simulink model "final63level"  (R2020a)
settings: Solver=ode45  StartTime=0.0  StopTime=.05  RelTol=5e-7  EnableMultiTasking=on
libraries: powerlib x42, re_lib x1, powerlib_meascontrol x1
settings Model: Creator=harish  LastModifiedBy=sunil
settings SolverCC: AlgebraicLoopSolver=LineSearch
settings DataIOCC: LimitDataPoints=on  SaveFormat=Array  ReturnWorkspaceOutputs=off
settings OptimizationCC: LifeSpan=inf
settings DebuggingCC: SFUnexpectedBacktrackingDiag=warning  SFNoUnconditionalDefaultTransitionDiag=warning  SFExecutionAtInitializationDiag=none  ArithmeticOperatorsInVariantConditions=warning
settings HardwareCC: ProdBitPerPointer=32  ProdBitPerSizeT=32  ProdBitPerPtrDiffT=32  ProdLargestAtomicFloat=None  ProdIntDivRoundTo=Undefined  ProdEndianess=Unspecified  ProdWordSize=32  ProdHWDeviceType=32-bit Generic
settings ModelReferenceCC: PropagateSignalLabelsOutOfModel=off
settings SFSimCC: SimUseLocalCustomCode=off  CustomCodeUndefinedFunction=UseInterfaceOnly
settings RTWCC: RTWUseLocalCustomCode=off
settings CodeAppCC: StateflowObjectComments=on
settings GRTTargetCC: TargetLangStandard=C89/C90 (ANSI)
settings ConfigComp: CovMetricSettings=dw  CovHtmlReporting=on  CovSaveCumulativeToWorkspaceVar=on  CovSaveSingleToWorkspaceVar=on  CovExternalEMLEnable=off
settings SimscapeCC: SimscapeNormalizeSystem=off

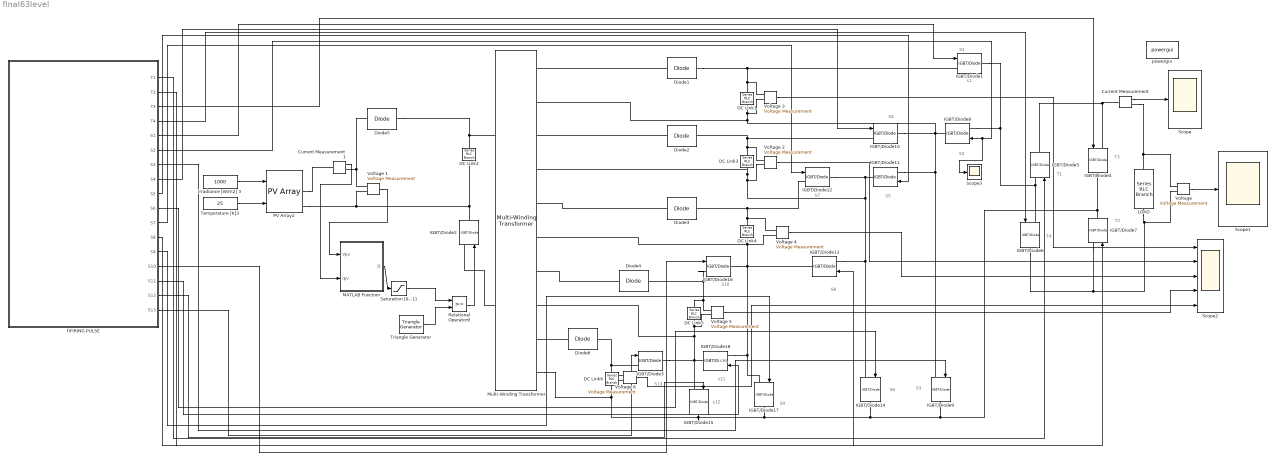
== system final63level ==
  note: s11
  note: s1
  note: S13
  note: s12
  note: s11
  note: S4
  note: S10
  note: S9
  note: S8
  note: S7
  note: S6
  note: S5
  note: S3
  note: S2
  note: S1
  note: T4
  note: T3
  note: T2
  note: T1
  Current Measurement : powerlib/Measurements/Current Measurement  PhasorSimulation=off  OutputType=Complex  PSBequivalent=0
  Current Measurement1 : powerlib/Measurements/Current Measurement  PhasorSimulation=off  OutputType=Complex  PSBequivalent=0
  DC Link1 : powerlib/Elements/Series RLC Branch  LConnTagsString=__new0  RConnTagsString=__new0  BranchType=C  Resistance=1.0  Inductance=1.0  SetiL0=off  InitialCurrent=0  Capacitance=3000e-6  Setx0=off  InitialVoltage=240/31  Measurements=None
      settings: SourceProductBaseCode=MT,PS
  DC Link2 : powerlib/Elements/Series RLC Branch  LConnTagsString=__new0  RConnTagsString=__new0  BranchType=C  Resistance=1.0  Inductance=1.0  SetiL0=off  InitialCurrent=0  Capacitance=300e+6  Setx0=on  InitialVoltage=256  Measurements=None
      settings: SourceProductBaseCode=MT,PS
  DC Link3 : powerlib/Elements/Series RLC Branch  LConnTagsString=__new0  RConnTagsString=__new0  BranchType=C  Resistance=1.0  Inductance=1.0  SetiL0=off  InitialCurrent=0  Capacitance=3000e-6  Setx0=off  InitialVoltage=32  Measurements=None
      settings: SourceProductBaseCode=MT,PS
  DC Link4 : powerlib/Elements/Series RLC Branch  LConnTagsString=__new0  RConnTagsString=__new0  BranchType=C  Resistance=1.0  Inductance=1.0  SetiL0=off  InitialCurrent=0  Capacitance=3000e-6  Setx0=off  InitialVoltage=68  Measurements=None
      settings: SourceProductBaseCode=MT,PS
  DC Link5 : powerlib/Elements/Series RLC Branch  LConnTagsString=__new0  RConnTagsString=__new0  BranchType=C  Resistance=1.0  Inductance=1.0  SetiL0=off  InitialCurrent=0  Capacitance=3000e-6  Setx0=off  InitialVoltage=128  Measurements=None
      settings: SourceProductBaseCode=MT,PS
  DC Link6 : powerlib/Elements/Series RLC Branch  LConnTagsString=__new0  RConnTagsString=__new0  BranchType=C  Resistance=1.0  Inductance=1.0  SetiL0=off  InitialCurrent=0  Capacitance=3000e-6  Setx0=off  InitialVoltage=128  Measurements=None
      settings: SourceProductBaseCode=MT,PS
  Diode{1..6} (6 alike) : powerlib/Power Electronics/Diode  Ron=0.001  Lon=0  Vf=0.8  IC=0  UseSnubber=0  Rs=500  Cs=250e-9  Measurements=off
  IGBT/Diode{1..18} (18 alike) : powerlib/Power Electronics/IGBT//Diode  Ron=1e-3  Rs=1e5  Cs=inf  Measurements=off
  Irradiance [W/m2] 3 : Constant  Value=1000
  LOAD : powerlib/Elements/Series RLC Branch  LConnTagsString=__new0  RConnTagsString=__new0  BranchType=RL  Resistance=250  Inductance=1e-3  SetiL0=off  InitialCurrent=0  Capacitance=1e-6  Setx0=off  InitialVoltage=0  Measurements=None
  MATLAB Function : MATLAB Function  TreatAsAtomicUnit=on
  Multi-Winding Transformer : powerlib/Elements/Multi-Winding Transformer  LeftWindings=1  RightWindings=5  TappedWindings=no taps  NumberOfTaps=4  SetSaturation=off  Hysteresis=off  DataFile='hysteresis.mat'  Measurements=None  UNITS=pu  NominalPower=[1000 10000]  NominalVoltages="[256 240/31   240*2/31   240*4/31  240*8/31  240*16/31]"  WindingResistances=[0 0 0 0 0 0]  WindingInductances="[0 0 0 0 0  0]"  Rm=0.11642  Lm=4.5959e+08  Saturation=[0 0;1.25e-06 1.44e+06;0.00052081 1.824e+06]  BreakLoop=off  DiscreteSolver=Trapezoidal iterative  DataType=off  InitialFlux=0  TransfoNumber=1
      settings: SourceProductBaseCode=PS
  PV Array2 : re_lib/Solar/PV Array  Npar=1  Nser=8  PlotType=array @ 1000 W/m2 & specified temperatures  S_vec="[ 1000  500  100 ]"  Temp_C_vec="[25  ]"  ModuleName=User-defined  PlotWhenSelected=off  Pm=213.15  Ncell=100  Voc=36.3  Isc=7.84  Vm=29  Im=7.35  beta_Voc_pc=-0.36099  alpha_Isc_pc=0.102  beta_Voc=-0.13104  alpha_Isc=0.0079968  IL=7.8541  I0=2.8969e-10  nI=0.58844  Rsh=372.6956  Rs=0.3942  RobustModel=off  RobustCellTemperature=25  BAL=on  Tc=1e-6  Tfilter=5e-5
  Relational Operator9 : RelationalOperator  OutDataTypeStr=boolean  RndMeth=Nearest
  Saturation [0...1] : Saturate  UpperLimit=1  LowerLimit=0
  Scope : Scope
  Scope1 : Scope
  Scope2 : Scope  NumInputPorts=5
  Scope3 : Scope
  Temperature [K]3 : Constant  Value=25
  Triangle Generator : powerlib_meascontrol/Pulse & Signal Generators/Triangle Generator  Freq=1e3  Phase=0  Ts=0
  Voltage {,1..6} (7 alike) : powerlib/Measurements/Voltage Measurement  PhasorSimulation=off  OutputType=Complex  PSBequivalent=0
  fiFIRING PULSE : Subsystem
  powergui : powerlib/powergui  Priority=1  SimulationMode=Discrete  SampleTime=5e-6  frequency=60  Iterations=50  frequencyindice=0  Pbase=100e6  ErrMax=1e-4  UnitsV=kV  UnitsW=MW  buscounter=0  FunctionMessages=off  echomessages=off  EnableUseOfTLC=off  CurrentSourceSwitches=on  DisableSnubberDevices=off  DisableRonSwitches=off  DisableVfSwitches=off  DisplayEquations=off  AutomaticDiscreteSolvers=off  SolverType=Tustin/Backward Euler (TBE)  Interpol=off  ExternalGateDelay=off  methode=off  Ts=100  x0status=blocks  SPID=off  SwTol=0  HookPort=off  NonlinearTolerance=1e-4  nMaxIteration=100  ContinueOnMaxIteration=off  RestoreLinks=warning  ResistiveCurrentMeasurement=off  Frange=[0:2:500]  Ylog=off  Xlog=on  ShowGrid=off  save=off  variable=ZData  structure=load  ZoomFFT=off  StartTime=0.0  cycles=1  DisplayStyle=1  fundamental=50  FreqAxis=on  MaxFrequency=1000  frequencyindicesteady=1  RmsSteady=1  display=off
  wires:
  "Voltage "/1 -> Scope1/1
  Current Measurement/1 -> Scope/1
  fiFIRING PULSE/1(T1) -> IGBT/Diode5/1
  fiFIRING PULSE/2(T2) -> IGBT/Diode7/1
  fiFIRING PULSE/3(T3) -> IGBT/Diode4/1
  fiFIRING PULSE/4(T4) -> IGBT/Diode6/1
  fiFIRING PULSE/5(S1) -> IGBT/Diode1/1
  fiFIRING PULSE/6(S2) -> Scope3/1, IGBT/Diode8/1
  fiFIRING PULSE/7(S3) -> IGBT/Diode9/1
  fiFIRING PULSE/8(S4) -> IGBT/Diode10/1
  fiFIRING PULSE/9(S5) -> IGBT/Diode11/1
  fiFIRING PULSE/10(S6) -> IGBT/Diode14/1
  fiFIRING PULSE/11(S7) -> IGBT/Diode12/1
  fiFIRING PULSE/12(S8) -> IGBT/Diode13/1
  fiFIRING PULSE/13(S9) -> IGBT/Diode17/1
  fiFIRING PULSE/14(S10) -> IGBT/Diode16/1
  MATLAB Function/1(D) -> Saturation [0...1]/1
  Voltage 1/1 -> MATLAB Function/1(Vpv)
  Current Measurement1/1 -> MATLAB Function/2(Ipv)
  Voltage 2/1 -> Scope2/2
  Voltage 3/1 -> Scope2/1
  Voltage 4/1 -> Scope2/3
  Voltage 5/1 -> Scope2/4
  Triangle Generator/1 -> Relational Operator9/2
  Relational Operator9/1 -> IGBT/Diode2/1
  Saturation [0...1]/1 -> Relational Operator9/1
  fiFIRING PULSE/17(S13) -> IGBT/Diode3/1
  fiFIRING PULSE/16(S12) -> IGBT/Diode15/1
  fiFIRING PULSE/15(S11) -> IGBT/Diode18/1
  Voltage 6/1 -> Scope2/5
  Temperature [K]3/1 -> PV Array2/2
  Irradiance [W/m2] 3/1 -> PV Array2/1
  connections:
  IGBT/Diode4/LConn1 -- Current Measurement/LConn1 -- IGBT/Diode5/RConn1
  IGBT/Diode6/LConn1 -- IGBT/Diode8/LConn1 -- IGBT/Diode1/RConn1 -- IGBT/Diode5/LConn1
  "Voltage "/LConn2 -- LOAD/LConn1 -- IGBT/Diode6/RConn1 -- IGBT/Diode7/LConn1
  LOAD/RConn1 -- Current Measurement/RConn1 -- "Voltage "/LConn1
  IGBT/Diode8/RConn1 -- IGBT/Diode10/RConn1 -- IGBT/Diode11/LConn1 -- IGBT/Diode9/LConn1 -- Multi-Winding Transformer/RConn2 -- Voltage 3/LConn2 -- DC Link1/RConn1
  IGBT/Diode12/RConn1 -- IGBT/Diode14/LConn1 -- IGBT/Diode13/LConn1 -- Voltage 2/LConn2 -- DC Link3/RConn1 -- Multi-Winding Transformer/RConn4 -- IGBT/Diode11/RConn1
  IGBT/Diode13/RConn1 -- IGBT/Diode17/LConn1 -- IGBT/Diode18/LConn1 -- IGBT/Diode16/RConn1 -- Voltage 4/LConn2 -- DC Link4/RConn1 -- Multi-Winding Transformer/RConn6
  Voltage 5/LConn2 -- IGBT/Diode3/RConn1 -- IGBT/Diode15/LConn1 -- IGBT/Diode18/RConn1 -- Multi-Winding Transformer/RConn8 -- DC Link5/RConn1
  DC Link1/LConn1 -- IGBT/Diode1/LConn1 -- Diode1/RConn1 -- Voltage 3/LConn1
  Diode1/LConn1 -- Multi-Winding Transformer/RConn1
  Diode2/LConn1 -- Multi-Winding Transformer/RConn3
  Diode3/LConn1 -- Multi-Winding Transformer/RConn5
  Diode4/LConn1 -- Multi-Winding Transformer/RConn7
  Diode5/RConn1 -- Multi-Winding Transformer/LConn1 -- DC Link2/LConn1
  IGBT/Diode2/RConn1 -- PV Array2/RConn2 -- Voltage 1/LConn2 -- DC Link2/RConn1
  PV Array2/RConn1 -- Current Measurement1/LConn1
  Voltage 1/LConn1 -- Diode5/LConn1 -- Current Measurement1/RConn1
  IGBT/Diode10/LConn1 -- Diode2/RConn1 -- Voltage 2/LConn1 -- DC Link3/LConn1
  Voltage 4/LConn1 -- DC Link4/LConn1 -- Diode3/RConn1 -- IGBT/Diode12/LConn1
  IGBT/Diode16/LConn1 -- Diode4/RConn1 -- DC Link5/LConn1 -- Voltage 5/LConn1
  Multi-Winding Transformer/LConn2 -- IGBT/Diode2/LConn1
  Diode6/LConn1 -- Multi-Winding Transformer/RConn9
  DC Link6/LConn1 -- Voltage 6/LConn1 -- IGBT/Diode3/LConn1 -- Diode6/RConn1
  IGBT/Diode14/RConn1 -- IGBT/Diode4/RConn1 -- IGBT/Diode7/RConn1 -- IGBT/Diode9/RConn1 -- Voltage 6/LConn2 -- DC Link6/RConn1 -- Multi-Winding Transformer/RConn10 -- IGBT/Diode15/RConn1 -- IGBT/Diode17/RConn1

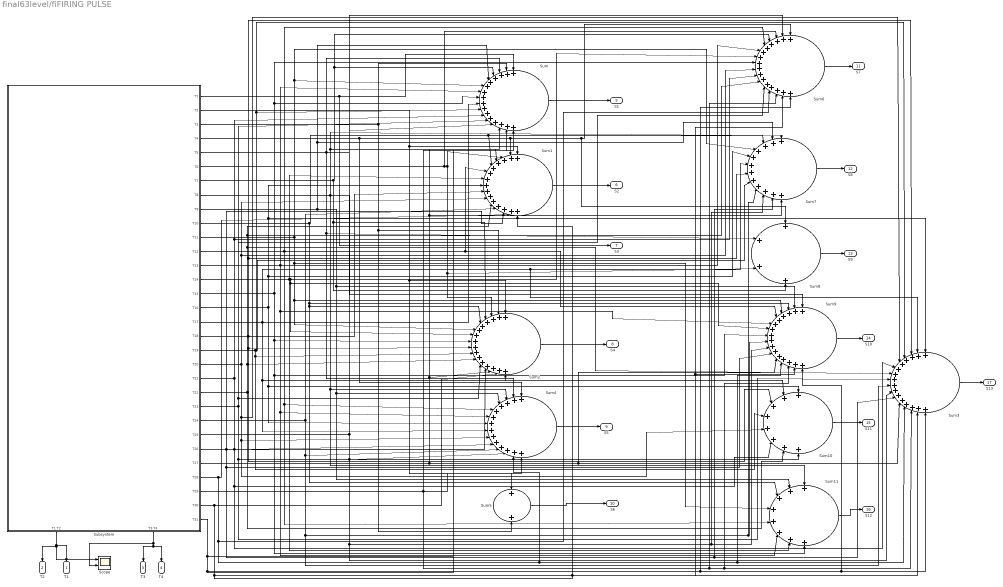
== system final63level/fiFIRING PULSE ==
  Scope : Scope  NumInputPorts=2
  Subsystem : Subsystem
      settings: PortSchema="{\"entries\":[{\"content\":{\"sides\":[{\"content\":{\"connectorIds\":[]},\"type\":\"ConnectorPlacement.EquallySpacedRectSide\",\"uuid\":\"70ad2b70-9561-48a4-a77f-34076edeb7a4\"},{\"content\":{\"connectorIds\":[\"Out1\",\"Out2\",\"Out3\",\"Out4\",\"Out5\",\"Out6\",\"Out7\",\"Out8\",\"Out9\",\"Out10\",\"Out11\",\"Out12\",\"Out13\",\"Out14\",\"Out15\",\"Out16\",\"Out17\",\"Out18\",\"Out19\",\"Out20\",\"Out21\",\"Out22\",\"Out23\",\"Out24\",\"Out25\",\"Out26\",\"Out27\",\"Out28\",\"Out29\",\"Out30\",\"Out31\"],\"side\":\"RIGHT\"},\"type\":\"ConnectorPlacement.EquallySpacedRectSide\",\"uuid\":\"b5d39657-1e04-4169-b553-b1962bf1f0e9\"},{\"content\":{\"connectorIds\":[],\"side\":\"TOP\"},\"type\":\"ConnectorPlacement.EquallySpacedRectSide\",\"uuid\":\"9b65afcb-07a6-4c10-8a50-7795185a824f\"},{\"content\":{\"connectorIds\":[\"Out32\",\"Out33\"],\"side\":\"BOTTOM\"},\"type\":\"ConnectorPlacement.EquallySpacedRectSide\",\"uuid\":\"1cd67243-db2c-4ba2-9ee1-558f28b37d25\"}]},\"type\":\"ConnectorPlacement.EquallySpacedConnector\",\"uuid\":\"3c7b11bc-dca1-47b6-888c-d1613d80d2b8\"}],\"packageUris\":[\"http://schema.mathworks.com/mf0/Connector/19700101\"],\"version\":\"1.0\"}"
  Sum{,2..3,6,9} (5 alike) : Sum  Inputs=++++++++++++++++
  Sum1 : Sum  Inputs=+++++++++++++++
  Sum10 : Sum  Inputs=++++++++
  Sum11 : Sum  Inputs=++++++++
  Sum4 : Sum  Inputs=++++++++++++++
  Sum5 : Sum
  Sum7 : Sum  Inputs=++++++++++++
  Sum8 : Sum  Inputs=++++
  T1 : Outport  VectorParamsAs1DForOutWhenUnconnected=off
  T2 : Outport  Port=2  VectorParamsAs1DForOutWhenUnconnected=off
  T3 : Outport  Port=3  VectorParamsAs1DForOutWhenUnconnected=off
  T4 : Outport  Port=4  VectorParamsAs1DForOutWhenUnconnected=off
  S1 : Outport  Port=5  VectorParamsAs1DForOutWhenUnconnected=off
  S2 : Outport  Port=6  VectorParamsAs1DForOutWhenUnconnected=off
  S3 : Outport  Port=7  VectorParamsAs1DForOutWhenUnconnected=off
  S4 : Outport  Port=8  VectorParamsAs1DForOutWhenUnconnected=off
  S5 : Outport  Port=9  VectorParamsAs1DForOutWhenUnconnected=off
  S6 : Outport  Port=10  VectorParamsAs1DForOutWhenUnconnected=off
  S7 : Outport  Port=11  VectorParamsAs1DForOutWhenUnconnected=off
  S8 : Outport  Port=12  VectorParamsAs1DForOutWhenUnconnected=off
  S9 : Outport  Port=13  VectorParamsAs1DForOutWhenUnconnected=off
  S10 : Outport  Port=14  VectorParamsAs1DForOutWhenUnconnected=off
  S11 : Outport  Port=15  VectorParamsAs1DForOutWhenUnconnected=off
  S12 : Outport  Port=16  VectorParamsAs1DForOutWhenUnconnected=off
  S13 : Outport  Port=17  VectorParamsAs1DForOutWhenUnconnected=off
  wires:
  Sum/1 -> S1/1
  Sum1/1 -> S2/1
  Sum2/1 -> S4/1
  Sum4/1 -> S5/1
  Sum5/1 -> S6/1
  Sum6/1 -> S7/1
  Sum7/1 -> S8/1
  Sum8/1 -> S9/1
  Sum9/1 -> S10/1
  Sum10/1 -> S11/1
  Sum11/1 -> S12/1
  Subsystem/1(T1) -> S3/1, Sum/1
  Sum3/1 -> S13/1
  Subsystem/2(T2) -> Sum5/1, Sum2/1, Sum1/1
  Subsystem/3(T3) -> Sum5/2, Sum2/2, Sum/2
  Subsystem/4(T4) -> Sum8/1, Sum6/1, Sum1/2, Sum4/1
  Subsystem/5(T5) -> Sum/3, Sum6/2, Sum4/2, Sum8/2
  Subsystem/6(T6) -> Sum6/3, Sum8/3, Sum2/3, Sum1/3
  Subsystem/7(T7) -> Sum2/4, Sum8/4, Sum6/4, Sum/4
  Subsystem/8(T8) -> Sum11/1, Sum4/3, Sum9/1, Sum7/1, Sum1/4
  Subsystem/9(T9) -> Sum7/2, Sum/5, Sum11/2, Sum4/4, Sum9/2
  Subsystem/10(T10) -> Sum1/5, Sum7/3, Sum11/3, Sum2/5, Sum9/3
  Subsystem/11(T11) -> Sum7/4, Sum/6, Sum2/6, Sum9/4, Sum11/4
  Subsystem/12(T12) -> Sum9/5, Sum1/6, Sum11/5, Sum4/5, Sum6/5
  Subsystem/13(T13) -> Sum11/6, Sum4/6, Sum9/6, Sum6/6, Sum/7
  Subsystem/14(T14) -> Sum2/7, Sum9/7, Sum6/7, Sum1/7, Sum11/7
  Subsystem/15(T15) -> Sum6/8, Sum/8, Sum9/8, Sum11/8, Sum2/8
  Subsystem/16(T16) -> Sum7/5, Sum1/8, Sum3/1, Sum4/7, Sum10/1
  Subsystem/17(T17) -> Sum3/2, Sum7/6, Sum4/8, Sum10/2, Sum/9
  Subsystem/18(T18) -> Sum3/3, Sum7/7, Sum10/3, Sum2/9, Sum1/9
  Subsystem/19(T19) -> Sum3/4, Sum/10, Sum7/8, Sum10/4, Sum2/10
  Subsystem/20(T20) -> Sum6/9, Sum1/10, Sum10/5, Sum4/9, Sum3/5
  Subsystem/21(T21) -> Sum/11, Sum6/10, Sum3/6, Sum10/6, Sum4/10
  Subsystem/22(T22) -> Sum1/11, Sum6/11, Sum3/7, Sum2/11, Sum10/7
  Subsystem/23(T23) -> Sum2/12, Sum/12, Sum6/12, Sum3/8, Sum10/8
  Subsystem/24(T24) -> Sum1/12, Sum4/11, Sum9/9, Sum7/9, Sum3/9
  Subsystem/25(T25) -> Sum3/10, Sum9/10, Sum7/10, Sum4/12, Sum/13
  Subsystem/26(T26) -> Sum1/13, Sum2/13, Sum3/11, Sum7/11, Sum9/11
  Subsystem/27(T27) -> Sum9/12, Sum3/12, Sum2/14, Sum7/12, Sum/14
  Subsystem/28(T28) -> Sum3/13, Sum9/13, Sum4/13, Sum6/13, Sum1/14
  Subsystem/29(T29) -> Sum9/14, Sum3/14, Sum6/14, Sum4/14, Sum/15
  Subsystem/30(T30) -> Sum2/15, Sum9/15, Sum6/15, Sum1/15, Sum3/15
  Subsystem/31(T31) -> Sum/16, Sum3/16, Sum9/16, Sum6/16, Sum2/16
  Subsystem/32(T1 T2) -> Scope/1, T2/1, T1/1
  Subsystem/33(T3 T4) -> Scope/2, T3/1, T4/1

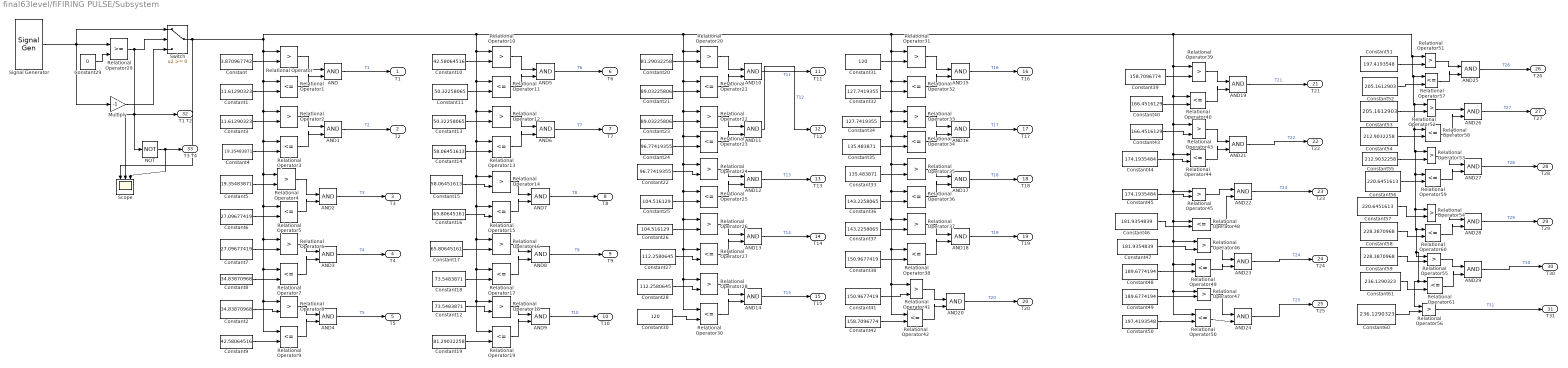
== system final63level/fiFIRING PULSE/Subsystem ==
  AND{,1..29} (30 alike) : Logic  IconShape=distinctive  AllPortsSameDT=off  OutDataTypeStr=boolean
  Constant : Constant  Value=3.870967742
  Constant1 : Constant  Value=11.61290323
  Constant10 : Constant  Value=42.58064516
  Constant11 : Constant  Value=50.32258065
  Constant12 : Constant  Value=73.5483871
  Constant13 : Constant  Value=50.32258065
  Constant14 : Constant  Value=58.06451613
  Constant15 : Constant  Value=58.06451613
  Constant16 : Constant  Value=65.80645161
  Constant17 : Constant  Value=65.80645161
  Constant18 : Constant  Value=73.5483871
  Constant19 : Constant  Value=81.29032258
  Constant2 : Constant  Value=34.83870968
  Constant20 : Constant  Value=81.29032258
  Constant21 : Constant  Value=89.03225806
  Constant22 : Constant  Value=96.77419355
  Constant23 : Constant  Value=89.03225806
  Constant24 : Constant  Value=96.77419355
  Constant25 : Constant  Value=104.516129
  Constant26 : Constant  Value=104.516129
  Constant27 : Constant  Value=112.2580645
  Constant28 : Constant  Value=112.2580645
  Constant29 : Constant  Value=0
  Constant3 : Constant  Value=11.61290323
  Constant30 : Constant  Value=120
  Constant31 : Constant  Value=120
  Constant32 : Constant  Value=127.7419355
  Constant33 : Constant  Value=135.483871
  Constant34 : Constant  Value=127.7419355
  Constant35 : Constant  Value=135.483871
  Constant36 : Constant  Value=143.2258065
  Constant37 : Constant  Value=143.2258065
  Constant38 : Constant  Value=150.9677419
  Constant39 : Constant  Value=158.7096774
  Constant4 : Constant  Value=19.35483871
  Constant40 : Constant  Value=166.4516129
  Constant41 : Constant  Value=150.9677419
  Constant42 : Constant  Value=158.7096774
  Constant43 : Constant  Value=166.4516129
  Constant44 : Constant  Value=174.1935484
  Constant45 : Constant  Value=174.1935484
  Constant46 : Constant  Value=181.9354839
  Constant47 : Constant  Value=181.9354839
  Constant48 : Constant  Value=189.6774194
  Constant49 : Constant  Value=189.6774194
  Constant5 : Constant  Value=19.35483871
  Constant50 : Constant  Value=197.4193548
  Constant51 : Constant  Value=197.4193548
  Constant52 : Constant  Value=205.1612903
  Constant53 : Constant  Value=205.1612903
  Constant54 : Constant  Value=212.9032258
  Constant55 : Constant  Value=212.9032258
  Constant56 : Constant  Value=220.6451613
  Constant57 : Constant  Value=220.6451613
  Constant58 : Constant  Value=228.3870968
  Constant59 : Constant  Value=228.3870968
  Constant6 : Constant  Value=27.09677419
  Constant60 : Constant  Value=236.1290323
  Constant61 : Constant  Value=236.1290323
  Constant7 : Constant  Value=27.09677419
  Constant8 : Constant  Value=34.83870968
  Constant9 : Constant  Value=42.58064516
  Multiply : Gain  Gain=-1
  NOT : Logic  Operator=NOT  IconShape=distinctive  AllPortsSameDT=off  OutDataTypeStr=boolean
  Relational Operator{,2,4,6,8,10,12,14,16,18,20,22,24,26,28,31,33,35,37,39,41,43,45..47,51..56} (31 alike) : RelationalOperator  Operator=>  OutDataTypeStr=boolean  RndMeth=Nearest
  Relational Operator{1,3,5,7,9,11,13,15,17,19,21,23,25,27,30,32,34,36,38,40,42,44,48..50,57..61} (30 alike) : RelationalOperator  Operator=<=  OutDataTypeStr=boolean  RndMeth=Nearest
  Relational Operator29 : RelationalOperator  OutDataTypeStr=boolean  RndMeth=Nearest
  Scope : Scope  NumInputPorts=3
  Signal Generator : SignalGenerator  Amplitude=240  Frequency=50
  Switch : Switch
  T1 : Outport
  T2 : Outport  Port=2
  T3 : Outport  Port=3
  T4 : Outport  Port=4
  T5 : Outport  Port=5
  T6 : Outport  Port=6
  T7 : Outport  Port=7
  T8 : Outport  Port=8
  T9 : Outport  Port=9
  T10 : Outport  Port=10
  T11 : Outport  Port=11
  T12 : Outport  Port=12
  T13 : Outport  Port=13
  T14 : Outport  Port=14
  T15 : Outport  Port=15
  T16 : Outport  Port=16
  T17 : Outport  Port=17
  T18 : Outport  Port=18
  T19 : Outport  Port=19
  T20 : Outport  Port=20
  T21 : Outport  Port=21
  T22 : Outport  Port=22
  T23 : Outport  Port=23
  T24 : Outport  Port=24
  T25 : Outport  Port=25
  T26 : Outport  Port=26
  T27 : Outport  Port=27
  T28 : Outport  Port=28
  T29 : Outport  Port=29
  T30 : Outport  Port=30
  T31 : Outport  Port=31
  T1 T2 : Outport  Port=32
  T3 T4 : Outport  Port=33
  wires:
  Relational Operator52/1 -> AND26/1
  Relational Operator7/1 -> AND3/2
  AND24/1 -> T25/1  "T25"
  Relational Operator55/1 -> AND29/1
  Signal Generator/1 -> Multiply/1, Switch/1, Relational Operator29/1
  AND19/1 -> T21/1  "T21"
  Constant21/1 -> Relational Operator21/2
  AND/1 -> T1/1  "T1"
  Constant36/1 -> Relational Operator36/2
  AND25/1 -> T26/1  "T26"
  Constant49/1 -> Relational Operator47/2
  Constant33/1 -> Relational Operator35/2
  Relational Operator29/1 -> Switch/2, T1 T2/1, Scope/2, NOT/1
  Relational Operator31/1 -> AND15/1
  Constant13/1 -> Relational Operator12/2
  AND29/1 -> T30/1  "T30"
  AND8/1 -> T9/1  "T9"
  Relational Operator44/1 -> AND21/2
  Constant1/1 -> Relational Operator1/2
  AND28/1 -> T29/1  "T29"
  Constant/1 -> Relational Operator/2
  Constant58/1 -> Relational Operator60/2
  Constant10/1 -> Relational Operator10/2
  Constant19/1 -> Relational Operator19/2
  Constant48/1 -> Relational Operator49/2
  Constant57/1 -> Relational Operator54/2
  Relational Operator43/1 -> AND21/1
  Relational Operator54/1 -> AND28/1
  Relational Operator34/1 -> AND16/2
  Relational Operator16/1 -> AND8/1
  Relational Operator9/1 -> AND4/2
  AND23/1 -> T24/1  "T24"
  AND22/1 -> T23/1  "T23"
  Constant52/1 -> Relational Operator57/2
  Relational Operator5/1 -> AND2/2
  AND4/1 -> T5/1  "T5"
  AND26/1 -> T27/1  "T27"
  Constant25/1 -> Relational Operator25/2
  Relational Operator35/1 -> AND17/1
  Constant11/1 -> Relational Operator11/2
  Constant41/1 -> Relational Operator41/2
  Constant29/1 -> Relational Operator29/2
  Relational Operator23/1 -> AND11/2
  Relational Operator47/1 -> AND24/1
  Relational Operator37/1 -> AND18/1
  AND17/1 -> T18/1  "T18"
  Relational Operator60/1 -> AND28/2
  Constant43/1 -> Relational Operator43/2
  Relational Operator15/1 -> AND7/2
  Relational Operator59/1 -> AND27/2
  AND2/1 -> T3/1  "T3"
  Constant51/1 -> Relational Operator51/2
  Constant32/1 -> Relational Operator32/2
  AND11/1 -> T12/1  "T12"
  Constant9/1 -> Relational Operator9/2
  Relational Operator10/1 -> AND5/1
  Relational Operator49/1 -> AND23/2
  Constant27/1 -> Relational Operator27/2
  Constant38/1 -> Relational Operator38/2
  Constant31/1 -> Relational Operator31/2
  Relational Operator57/1 -> AND25/2
  Relational Operator51/1 -> AND25/1
  Constant53/1 -> Relational Operator52/2
  AND27/1 -> T28/1  "T28"
  AND6/1 -> T7/1  "T7"
  Relational Operator8/1 -> AND4/1
  Relational Operator45/1 -> AND22/1
  Constant55/1 -> Relational Operator53/2
  Relational Operator1/1 -> AND/2
  AND21/1 -> T22/1  "T22"
  Constant56/1 -> Relational Operator59/2
  Constant54/1 -> Relational Operator58/2
  Relational Operator11/1 -> AND5/2
  Relational Operator3/1 -> AND1/2
  Relational Operator26/1 -> AND13/1
  AND12/1 -> T13/1  "T13"
  Relational Operator20/1 -> AND10/1
  Relational Operator2/1 -> AND1/1
  Constant5/1 -> Relational Operator4/2
  Constant37/1 -> Relational Operator37/2
  Relational Operator22/1 -> AND11/1
  Constant20/1 -> Relational Operator20/2
  Constant40/1 -> Relational Operator40/2
  Constant26/1 -> Relational Operator26/2
  Relational Operator46/1 -> AND23/1
  Relational Operator39/1 -> AND19/1
  Relational Operator38/1 -> AND18/2
  Relational Operator50/1 -> AND24/2
  Constant22/1 -> Relational Operator24/2
  AND14/1 -> T15/1  "T15"
  Constant46/1 -> Relational Operator48/2
  Constant45/1 -> Relational Operator45/2
  Relational Operator41/1 -> AND20/1
  Constant39/1 -> Relational Operator39/2
  Multiply/1 -> Switch/3
  Relational Operator4/1 -> AND2/1
  Constant44/1 -> Relational Operator44/2
  Relational Operator48/1 -> AND22/2
  Relational Operator42/1 -> AND20/2
  Constant50/1 -> Relational Operator50/2
  Constant47/1 -> Relational Operator46/2
  Relational Operator24/1 -> AND12/1
  AND16/1 -> T17/1  "T17"
  Constant35/1 -> Relational Operator34/2
  AND10/1 -> T11/1  "T11"
  AND9/1 -> T10/1  "T10"
  Relational Operator21/1 -> AND10/2
  Constant42/1 -> Relational Operator42/2
  AND15/1 -> T16/1  "T16"
  Relational Operator40/1 -> AND19/2
  NOT/1 -> T3 T4/1, Scope/3
  Relational Operator58/1 -> AND26/2
  Relational Operator12/1 -> AND6/1
  Constant16/1 -> Relational Operator15/2
  Relational Operator30/1 -> AND14/2
  Relational Operator32/1 -> AND15/2
  AND20/1 -> T20/1  "T20"
  Constant30/1 -> Relational Operator30/2
  AND18/1 -> T19/1  "T19"
  Constant28/1 -> Relational Operator28/2
  Relational Operator28/1 -> AND14/1
  Relational Operator27/1 -> AND13/2
  Constant15/1 -> Relational Operator14/2
  AND5/1 -> T6/1  "T6"
  Constant18/1 -> Relational Operator17/2
  Constant14/1 -> Relational Operator13/2
  AND1/1 -> T2/1  "T2"
  Constant6/1 -> Relational Operator5/2
  AND13/1 -> T14/1  "T14"
  Constant34/1 -> Relational Operator33/2
  Relational Operator14/1 -> AND7/1
  Relational Operator17/1 -> AND8/2
  Constant2/1 -> Relational Operator8/2
  Relational Operator33/1 -> AND16/1
  Relational Operator19/1 -> AND9/2
  Relational Operator6/1 -> AND3/1
  AND7/1 -> T8/1  "T8"
  Constant17/1 -> Relational Operator16/2
  Relational Operator18/1 -> AND9/1
  Constant24/1 -> Relational Operator23/2
  Relational Operator36/1 -> AND17/2
  Constant23/1 -> Relational Operator22/2
  Relational Operator13/1 -> AND6/2
  Relational Operator53/1 -> AND27/1
  Constant8/1 -> Relational Operator7/2
  Relational Operator/1 -> AND/1
  Constant3/1 -> Relational Operator2/2
  AND3/1 -> T4/1  "T4"
  Relational Operator25/1 -> AND12/2
  Constant12/1 -> Relational Operator18/2
  Constant4/1 -> Relational Operator3/2
  Constant7/1 -> Relational Operator6/2
  Constant59/1 -> Relational Operator55/2
  Switch/1 -> Relational Operator39/1, Relational Operator43/1, Relational Operator45/1, Relational Operator48/1, Relational Operator46/1, Relational Operator49/1, Relational Operator47/1, Relational Operator50/1, Relational Operator44/1, Relational Operator40/1, Relational Operator58/1, Relational Operator56/1, Relational Operator61/1, Relational Operator55/1, Relational Operator60/1, Relational Operator54/1, Relational Operator59/1, Relational Operator53/1, Relational Operator52/1, Relational Operator57/1, Relational Operator51/1, Relational Operator31/1, Relational Operator33/1, Relational Operator35/1, Relational Operator37/1, Relational Operator38/1, Relational Operator41/1, Relational Operator42/1, Relational Operator36/1, Relational Operator34/1, Relational Operator32/1, Relational Operator20/1, Relational Operator22/1, Relational Operator24/1, Relational Operator26/1, Relational Operator28/1, Relational Operator30/1, Relational Operator27/1, Relational Operator25/1, Relational Operator23/1, Relational Operator21/1, Relational Operator10/1, Relational Operator12/1, Relational Operator18/1, Relational Operator19/1, Relational Operator17/1, Relational Operator16/1, Relational Operator15/1, Relational Operator14/1, Relational Operator13/1, Relational Operator11/1, Relational Operator/1, Relational Operator2/1, Relational Operator8/1, Relational Operator9/1, Relational Operator7/1, Relational Operator6/1, Relational Operator5/1, Relational Operator4/1, Relational Operator3/1, Relational Operator1/1, Scope/1
  Relational Operator56/1 -> T31/1  "T31"
  Constant60/1 -> Relational Operator56/2
  Constant61/1 -> Relational Operator61/2
  Relational Operator61/1 -> AND29/2

== matlab function final63level/MATLAB Function ==
  settings: updateMethod=DISCRETE  sampleTime=1e-4
  data: Vpv input; D output; Ipv input
function D = PandO(Vpv,Ipv)
%#codegen
% ************************************************************
% MATLAB implementation of a Perturb and Observe algorithm
% for Maximum Power Point Tracking. This algorithm is designed
% to operate with a buck converter
%
% Created by: Carlos Osorio
% ************************************************************

% Define internal values for the voltage and power as persistent
% variables
persistent Dprev Pprev Vprev

% Initialize the internal values for the voltage and power on the
% first pass
if isempty(Dprev)
    Dprev = 0.9;
    Vprev = 256;
    Pprev = 2000;
end

% Initialize algorithm parameters
deltaD = 0.0025;

% Calculate measured array power
Ppv = Vpv*Ipv;

% Increase or decrease duty cycle based on conditions
if (Ppv-Pprev) ~= 0
    if (Ppv-Pprev) > 0
        if (Vpv-Vprev) > 0
            D = Dprev - deltaD;
        else
            D = Dprev + deltaD;
        end
    else
        if (Vpv-Vprev) > 0
            D = Dprev + deltaD;
        else
            D = Dprev - deltaD;
        end        
    end
else
    D = Dprev;
end

% Update internal values
Dprev = D;
Vprev = Vpv;
Pprev = Ppv;
